simulink model "Controle_de_Volume_Tanque"  (R2016a)
settings: Solver=ode45  StartTime=0.0  StopTime=inf  RelTol=1e-3
libraries: sh_lib x8, nesl_utility x7, fl_lib x4, simulink x2
settings Model: Creator=kreislerb  LastModifiedBy=kreislerb
settings DataIOCC: LimitDataPoints=on  SaveFormat=Array
settings HardwareCC: ProdBitPerPointer=32  ProdLargestAtomicFloat=None  ProdIntDivRoundTo=Undefined  ProdEndianess=Unspecified  ProdWordSize=32  ProdHWDeviceType=32-bit Generic
settings ModelReferenceCC: PropagateSignalLabelsOutOfModel=off
settings ConfigComp: CovModelRefEnable=Off

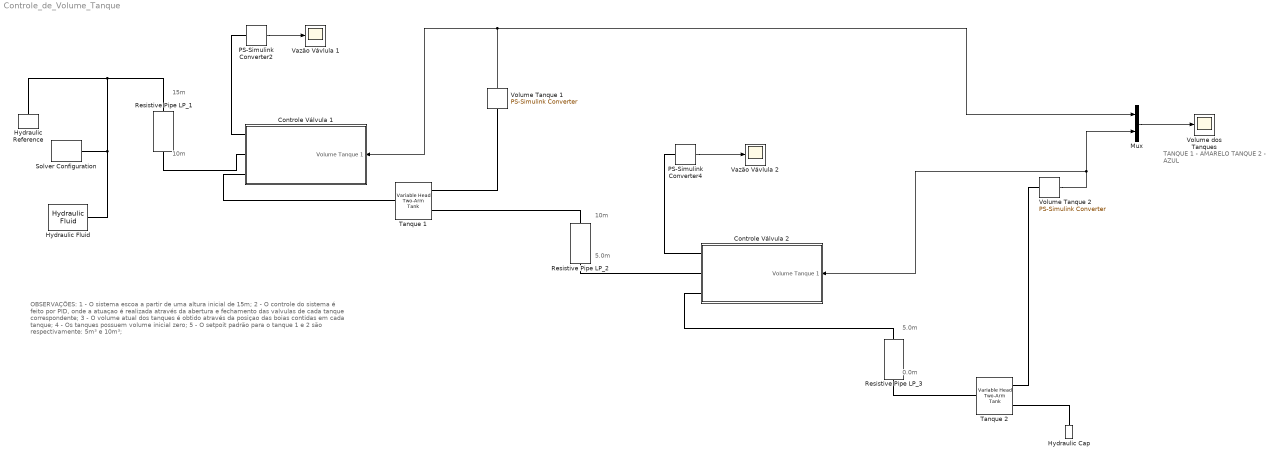
== system Controle_de_Volume_Tanque ==
  note: OBSERVAÇÕES:
      |
      | 1 - O sistema escoa a partir de uma altura inicial de 15m;
      | 2 - O controle do sistema é feito por PID, onde a atuaçao é realizada através da abertura e fechamento das valvulas de cada tanque correspondente;
      | 3 - O volume atual dos tanques é obtido através da posiçao das boias contidas em cada tanque;
      | 4 - Os tanques possuem volume inicial zero;
      | 5 - O setpoit padrão para o tanque 1 e 2 são respectivamente: 5m³ e 10m³;
  note: TANQUE 1 - AMARELO
      | TANQUE 2 - AZUL
  note: 10m
  note: 15m
  note: 10m
  note: 5.0m
  note: 5.0m
  note: 0.0m
  Controle Válvula 1 : Subsystem  mask{SetPoint=5}
  Controle Válvula 2 : Subsystem  mask{SetPoint=10}
  Hydraulic Cap : fl_lib/Hydraulic/Hydraulic Elements/Hydraulic Cap  p_specify=off  p_priority=High  p=0 Pa
  Hydraulic Fluid : sh_lib/Hydraulic Utilities/Hydraulic Fluid  DataSource=1  SelFluid=24  SysTemp=25  TrapAir=0.001  ViscDerFactor=1  range_error=2
  Hydraulic Reference : fl_lib/Hydraulic/Hydraulic Elements/Hydraulic Reference
  Mux : Mux  Inputs=2
  PS-Simulink Converter2 : nesl_utility/PS-Simulink Converter  PhysicalDomain=network_engine_domain  SubClassName=ps_output  LeftPortType=input  RightPortType=output  PseudoPeriodic=off  Frequencies=[]  Unit=m^3/s  AffineConversion=off
  PS-Simulink Converter4 : nesl_utility/PS-Simulink Converter  PhysicalDomain=network_engine_domain  SubClassName=ps_output  LeftPortType=input  RightPortType=output  PseudoPeriodic=off  Frequencies=[]  Unit=m^3/s  AffineConversion=off
  Resistive Pipe LP_1 : sh_lib/Low-Pressure Blocks/Resistive Pipe LP  cs_type=1  d_in=20 mm  area=1e-04 m^2  D_h=0.0112 m  s_factor=64  length=10 m  length_ad=1 m  roughness=0.005 mm  Re_lam=2e+03  Re_turb=4e+03  elevation_A=25 m  elevation_B=15 m
  Resistive Pipe LP_2 : sh_lib/Low-Pressure Blocks/Resistive Pipe LP  cs_type=1  d_in=20 mm  area=1e-04 m^2  D_h=0.0112 m  s_factor=64  length=5 m  length_ad=1 m  roughness=0.005 mm  Re_lam=2e+03  Re_turb=4e+03  elevation_A=10 m  elevation_B=5 m
  Resistive Pipe LP_3 : sh_lib/Low-Pressure Blocks/Resistive Pipe LP  cs_type=1  d_in=20 mm  area=1e-04 m^2  D_h=0.0112 m  s_factor=64  length=5 m  length_ad=1 m  roughness=0.005 mm  Re_lam=2e+03  Re_turb=4e+03  elevation_A=5 m  elevation_B=0 m
  Solver Configuration : nesl_utility/Solver Configuration  PhysicalDomain=network_engine_domain  SubClassName=solver  LeftPortType=input  RightPortType=generic  Accelerate=off  Tones=[]  Harmonics=[]  SimulateNoise=off  Profile=off  UseLocalSampling=off  EnableSwitchedLinearOptims=on  FrequencyDomain=off  UseCCode=off  RelTol=0.001  AbsTol=1e-06  MinStep=1e-09  ToWorkspace=off  RevertToSquareIcSolve=off  NumHomotopyIterations=100  PhasorMode=off  PhasorModeNumHarmonics=1  OverrideAbsTol=off  DoDC=off  ResidualTolerance=1e-09  UseLocalSolver=off  LocalSolverChoice=NE_BACKWARD_EULER_ADVANCER  LocalSolverSampleTime=0.001  DoFixedCost=off  MaxNonlinIter=3  MaxModeIter=2  LinearAlgebra=Full  DelaysMemoryBudget=1024  AutomaticFiltering=off  FilteringTimeConstant=0.001
  Tanque 1 : sh_lib/Low-Pressure Blocks/Variable Head Two-Arm Tank  init_volume=0 m^3  press=0 Pa  level_spec=1  tank_area=0.8 m^2  fluid_volume_tab=[ 0 0.0028 0.0065 0.0114 0.0176 0.0252 0.0344 0.0436 0.0512 0.0574 0.0623 0.066 0.0688 0.0707 0.07199999999999999 0.0727 ] m^3  fluid_level_tab=[ 0 0.02 0.04 0.06 0.08 0.1 0.12 0.14 0.16 0.18 0.2 0.22 0.24 0.26 0.28 0.3 ] m  pipe_diam_A=0.02 m  loss_coeff_A=1.2  pipe_diam_B=0.02 m  height_B=3 m  loss_coeff_B=1.2  interp_method=1  extrap_method=1
  Tanque 2 : sh_lib/Low-Pressure Blocks/Variable Head Two-Arm Tank  init_volume=0 m^3  press=0 Pa  level_spec=1  tank_area=0.8 m^2  fluid_volume_tab=[ 0 0.0028 0.0065 0.0114 0.0176 0.0252 0.0344 0.0436 0.0512 0.0574 0.0623 0.066 0.0688 0.0707 0.07199999999999999 0.0727 ] m^3  fluid_level_tab=[ 0 0.02 0.04 0.06 0.08 0.1 0.12 0.14 0.16 0.18 0.2 0.22 0.24 0.26 0.28 0.3 ] m  pipe_diam_A=0.02 m  loss_coeff_A=1.2  pipe_diam_B=0.01 m  height_B=0.5 m  loss_coeff_B=1.2  interp_method=1  extrap_method=1
  "Vazão Vávlula 1 " : Scope
  "Vazão Vávlula 2 " : Scope
  Volume Tanque 1 : nesl_utility/PS-Simulink Converter  PhysicalDomain=network_engine_domain  SubClassName=ps_output  LeftPortType=input  RightPortType=output  PseudoPeriodic=off  Frequencies=[]  Unit=m^3  AffineConversion=on
  Volume Tanque 2 : nesl_utility/PS-Simulink Converter  PhysicalDomain=network_engine_domain  SubClassName=ps_output  LeftPortType=input  RightPortType=output  PseudoPeriodic=off  Frequencies=[]  Unit=m^3  AffineConversion=on
  Volume dos Tanques : Scope
  wires:
  Mux/1 -> Volume dos Tanques/1
  Volume Tanque 1/1 -> Mux/1, Controle Válvula 1/1(Volume Tanque 1)
  Volume Tanque 2/1 -> Mux/2, Controle Válvula 2/1(Volume Tanque 1)
  PS-Simulink Converter2/1 -> "Vazão Vávlula 1 "/1
  PS-Simulink Converter4/1 -> "Vazão Vávlula 2 "/1
  connections:
  Tanque 1/RConn1 -- Volume Tanque 1/LConn1
  Solver Configuration/RConn1 -- Hydraulic Fluid/RConn1 -- Hydraulic Reference/LConn1 -- Resistive Pipe LP_1/LConn1
  Tanque 2/RConn1 -- Volume Tanque 2/LConn1
  Hydraulic Cap/LConn1 -- Tanque 2/RConn2
  Controle Válvula 1/RConn1 -- PS-Simulink Converter2/LConn1
  Controle Válvula 1/RConn2 -- Resistive Pipe LP_1/RConn1
  Controle Válvula 1/RConn3 -- Tanque 1/LConn1
  PS-Simulink Converter4/LConn1 -- Controle Válvula 2/RConn1
  Tanque 1/RConn2 -- Resistive Pipe LP_2/LConn1
  Resistive Pipe LP_2/RConn1 -- Controle Válvula 2/RConn2
  Controle Válvula 2/RConn3 -- Resistive Pipe LP_3/LConn1
  Resistive Pipe LP_3/RConn1 -- Tanque 2/LConn1

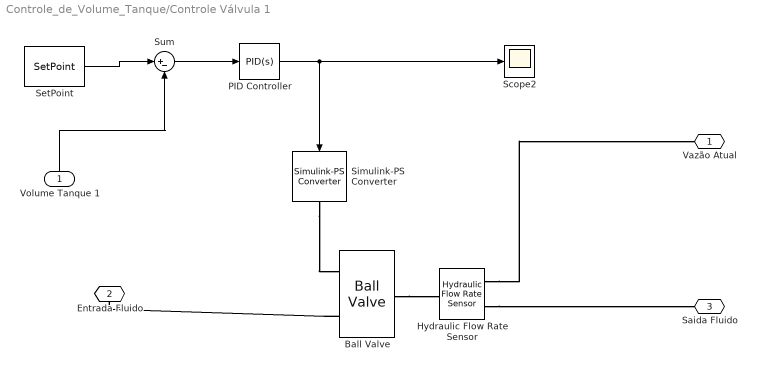
== system Controle_de_Volume_Tanque/Controle Válvula 1 ==
  Volume Tanque 1 : Inport
  Ball Valve : sh_lib/Valves/Flow Control Valves/Ball Valve  d_ball=0.1 m  d_orif=0.02 m  x_0=0 m  C_d=0.65  Re_cr=10  A_leak=1e-12 m^2
  Hydraulic Flow Rate Sensor : fl_lib/Hydraulic/Hydraulic Sensors/Hydraulic Flow Rate Sensor
  PID Controller : simulink/Continuous/PID Controller  Controller=PID  TimeDomain=Continuous-time  SampleTime=-1  IntegratorMethod=Forward Euler  FilterMethod=Forward Euler  Form=Parallel  UseFilter=on  ControllerParametersSource=internal  P=1000  I=0  D=0  N=100  InitialConditionSource=internal  InitialConditionForIntegrator=0  InitialConditionForFilter=0  ExternalReset=none  LimitOutput=off  UpperSaturationLimit=inf  LowerSaturationLimit=-inf  LinearizeAsGain=on  AntiWindupMode=none  Kb=1  TrackingMode=off  Kt=1  PParamMin=[]  PParamMax=[]  IParamMin=[]  IParamMax=[]  DParamMin=[]  DParamMax=[]  NParamMin=[]  NParamMax=[]  KbParamMin=[]  KbParamMax=[]  KtParamMin=[]  KtParamMax=[]  POutMin=[]  POutMax=[]  IOutMin=[]  IOutMax=[]  DOutMin=[]  DOutMax=[]  NOutMin=[]  NOutMax=[]  KbOutMin=[]  KbOutMax=[]  KtOutMin=[]  KtOutMax=[]  IntegratorOutMin=[]  IntegratorOutMax=[]  FilterOutMin=[]  FilterOutMax=[]  SumOutMin=[]  SumOutMax=[]  SumI1OutMin=[]  SumI1OutMax=[]  SumI2OutMin=[]  SumI2OutMax=[]  SumI3OutMin=[]  SumI3OutMax=[]  SumDOutMin=[]  SumDOutMax=[]  SaturationOutMin=[]  SaturationOutMax=[]  IntegratorContinuousStateAttributes=''  IntegratorStateMustResolveToSignalObject=off  IntegratorRTWStateStorageClass=Auto  FilterContinuousStateAttributes=''  FilterStateMustResolveToSignalObject=off  FilterRTWStateStorageClass=Auto  DifferentiatorICPrevScaledInput=0  DifferentiatorOutMin=[]  DifferentiatorOutMax=[]
  Scope2 : Scope
  SetPoint : Constant  Value=SetPoint
  Simulink-PS Converter : nesl_utility/Simulink-PS Converter  PhysicalDomain=network_engine_domain  SubClassName=ps_input  LeftPortType=input  RightPortType=output  PseudoPeriodic=off  Frequencies=[]  NoiseDistribution=none  NoiseParameters=[]  Unit=m  AffineConversion=off  InputFiltering=on  SimscapeFilterOrder=1  InputFilterTimeConstant=1  UdotUserProvided=2
  Sum : Sum  Inputs=|+-
  Vazão Atual : PMIOPort  Port=1  Side=Right
  Entrada Fluido : PMIOPort  Port=2  Side=Right
  Saida Fluido : PMIOPort  Port=3  Side=Right
  wires:
  Sum/1 -> PID Controller/1
  SetPoint/1 -> Sum/1
  PID Controller/1 -> Scope2/1, Simulink-PS Converter/1
  Volume Tanque 1/1 -> Sum/2
  connections:
  Hydraulic Flow Rate Sensor/RConn1 -- Vazão Atual/RConn1
  Ball Valve/LConn2 -- Entrada Fluido/RConn1
  Simulink-PS Converter/RConn1 -- Ball Valve/LConn1
  Ball Valve/RConn1 -- Hydraulic Flow Rate Sensor/LConn1
  Hydraulic Flow Rate Sensor/RConn2 -- Saida Fluido/RConn1

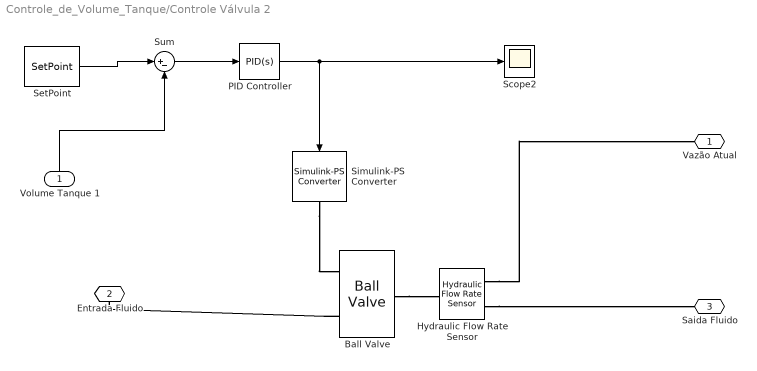
== system Controle_de_Volume_Tanque/Controle Válvula 2 ==
  Volume Tanque 1 : Inport
  Ball Valve : sh_lib/Valves/Flow Control Valves/Ball Valve  d_ball=0.1 m  d_orif=0.02 m  x_0=0 m  C_d=0.65  Re_cr=10  A_leak=1e-12 m^2
  Hydraulic Flow Rate Sensor : fl_lib/Hydraulic/Hydraulic Sensors/Hydraulic Flow Rate Sensor
  PID Controller : simulink/Continuous/PID Controller  Controller=PID  TimeDomain=Continuous-time  SampleTime=-1  IntegratorMethod=Forward Euler  FilterMethod=Forward Euler  Form=Parallel  UseFilter=on  ControllerParametersSource=internal  P=1000  I=0  D=0  N=100  InitialConditionSource=internal  InitialConditionForIntegrator=0  InitialConditionForFilter=0  ExternalReset=none  LimitOutput=off  UpperSaturationLimit=inf  LowerSaturationLimit=-inf  LinearizeAsGain=on  AntiWindupMode=none  Kb=1  TrackingMode=off  Kt=1  PParamMin=[]  PParamMax=[]  IParamMin=[]  IParamMax=[]  DParamMin=[]  DParamMax=[]  NParamMin=[]  NParamMax=[]  KbParamMin=[]  KbParamMax=[]  KtParamMin=[]  KtParamMax=[]  POutMin=[]  POutMax=[]  IOutMin=[]  IOutMax=[]  DOutMin=[]  DOutMax=[]  NOutMin=[]  NOutMax=[]  KbOutMin=[]  KbOutMax=[]  KtOutMin=[]  KtOutMax=[]  IntegratorOutMin=[]  IntegratorOutMax=[]  FilterOutMin=[]  FilterOutMax=[]  SumOutMin=[]  SumOutMax=[]  SumI1OutMin=[]  SumI1OutMax=[]  SumI2OutMin=[]  SumI2OutMax=[]  SumI3OutMin=[]  SumI3OutMax=[]  SumDOutMin=[]  SumDOutMax=[]  SaturationOutMin=[]  SaturationOutMax=[]  IntegratorContinuousStateAttributes=''  IntegratorStateMustResolveToSignalObject=off  IntegratorRTWStateStorageClass=Auto  FilterContinuousStateAttributes=''  FilterStateMustResolveToSignalObject=off  FilterRTWStateStorageClass=Auto  DifferentiatorICPrevScaledInput=0  DifferentiatorOutMin=[]  DifferentiatorOutMax=[]
  Scope2 : Scope
  SetPoint : Constant  Value=SetPoint
  Simulink-PS Converter : nesl_utility/Simulink-PS Converter  PhysicalDomain=network_engine_domain  SubClassName=ps_input  LeftPortType=input  RightPortType=output  PseudoPeriodic=off  Frequencies=[]  NoiseDistribution=none  NoiseParameters=[]  Unit=m  AffineConversion=off  InputFiltering=on  SimscapeFilterOrder=1  InputFilterTimeConstant=1  UdotUserProvided=2
  Sum : Sum  Inputs=|+-
  Vazão Atual : PMIOPort  Port=1  Side=Right
  Entrada Fluido : PMIOPort  Port=2  Side=Right
  Saida Fluido : PMIOPort  Port=3  Side=Right
  wires:
  Volume Tanque 1/1 -> Sum/2
  PID Controller/1 -> Simulink-PS Converter/1, Scope2/1
  SetPoint/1 -> Sum/1
  Sum/1 -> PID Controller/1
  connections:
  Hydraulic Flow Rate Sensor/RConn2 -- Saida Fluido/RConn1
  Ball Valve/RConn1 -- Hydraulic Flow Rate Sensor/LConn1
  Simulink-PS Converter/RConn1 -- Ball Valve/LConn1
  Ball Valve/LConn2 -- Entrada Fluido/RConn1
  Hydraulic Flow Rate Sensor/RConn1 -- Vazão Atual/RConn1
